simulink subsystem "encoder_velocidad"  (R2023b)
settings: Solver=VariableStepAuto  StartTime=0.0  StopTime=10.0  RelTol=1e-3
libraries: arduinosensorlib x2, simulink x1
settings Model: Creator=Usuario_UMA  LastModifiedBy=Manuel

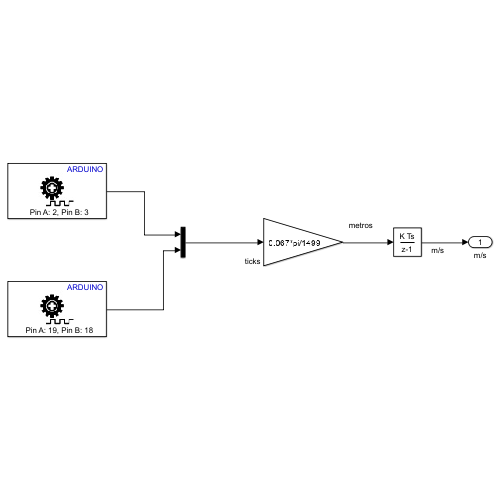
[thumbnail: Simulink's stored preview of the top-level diagram]
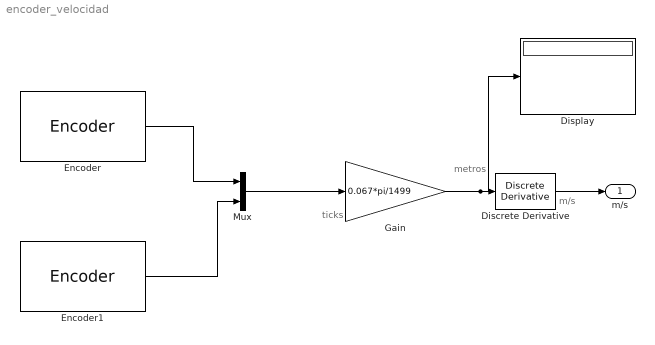
== system encoder_velocidad ==
  note: metros
  note: ticks
  note: m/s
  Discrete Derivative : simulink/Discrete/Discrete Derivative  gainval=1.0  ICPrevScaledInput=0.0  OutMin=[]  OutMax=[]  OutDataType=fixdt(1, 16)  OutScaling=2^-10  DoSatur=off
  Display : Display
  Encoder : arduinosensorlib/Encoder  InputA=2  InputB=3  Mode=No reset  SampleTime=-1
  Encoder1 : arduinosensorlib/Encoder  InputA=19  InputB=18  Mode=No reset  SampleTime=-1
  Gain : Gain  Gain=0.067*pi/1499  OutDataTypeStr=double
  Mux : Mux  Inputs=2
  m/s : Outport
  wires:
  Encoder/1 -> Mux/1
  Encoder1/1 -> Mux/2
  Mux/1 -> Gain/1
  Gain/1 -> Discrete Derivative/1, Display/1
  Discrete Derivative/1 -> m/s/1
